simulink model "vibration_absorber"  (R2020a)
settings: Solver=VariableStepAuto  StartTime=0.0  StopTime=10.0  RelTol=1e-3
PostLoadFcn:
  | M1=100;
  | K1=50;
  | b=50;
undefined symbols (not defined in the file): K12, M2
settings Model: Creator=Hp  LastModifiedBy=Hp

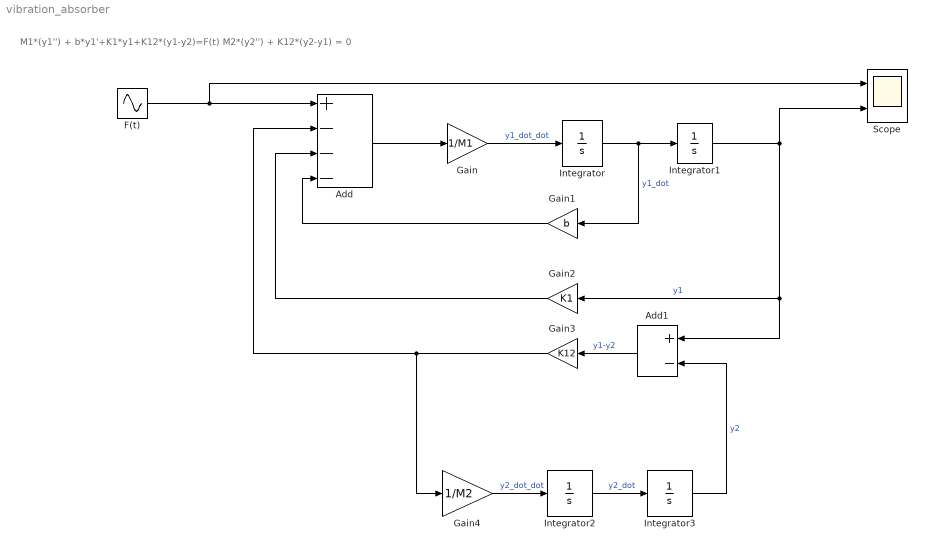
== system vibration_absorber ==
  note: M1*(y1'') + b*y1'+K1*y1+K12*(y1-y2)=F(t)
      | M2*(y2'') + K12*(y2-y1) = 0
  Add : Sum  Inputs=+---
  Add1 : Sum  Inputs=+-
  F(t) : Sin  Amplitude=2  Frequency=10  SampleTime=0.001
  Gain : Gain  Gain=1/M1
  Gain1 : Gain  Gain=b
  Gain2 : Gain  Gain=K1
  Gain3 : Gain  Gain=K12
  Gain4 : Gain  Gain=1/M2
  Integrator{,1..3} (4 alike) : Integrator
  Scope : Scope  NumInputPorts=2
  wires:
  Gain/1 -> Integrator/1  "y1_dot_dot"
  Integrator/1 -> Gain1/1, Integrator1/1  "y1_dot"
  Add/1 -> Gain/1
  F(t)/1 -> Scope/1, Add/1
  Integrator1/1 -> Gain2/1, Add1/1, Scope/2  "y1"
  Gain1/1 -> Add/4
  Gain2/1 -> Add/3
  Add1/1 -> Gain3/1  "y1-y2"
  Gain3/1 -> Gain4/1, Add/2
  Integrator2/1 -> Integrator3/1  "y2_dot"
  Gain4/1 -> Integrator2/1  "y2_dot_dot"
  Integrator3/1 -> Add1/2  "y2"
